simulink model "RuleBasedAlgo_sfunc_model"  (R2018b)
settings: Solver=ode2  StartTime=0.0  StopTime=inf  FixedStep=t_step  RelTol=1e-3
undefined symbols (not defined in the file or in its folder): A123_ESS, cs_ll, cs_ul
libraries: simulink x1
settings Model: Creator=Aman-Home  LastModifiedBy=Aman-Home

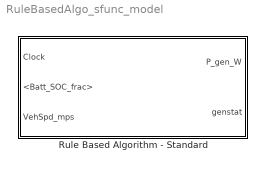
== system RuleBasedAlgo_sfunc_model ==
  Rule Based Algorithm - Standard : Subsystem

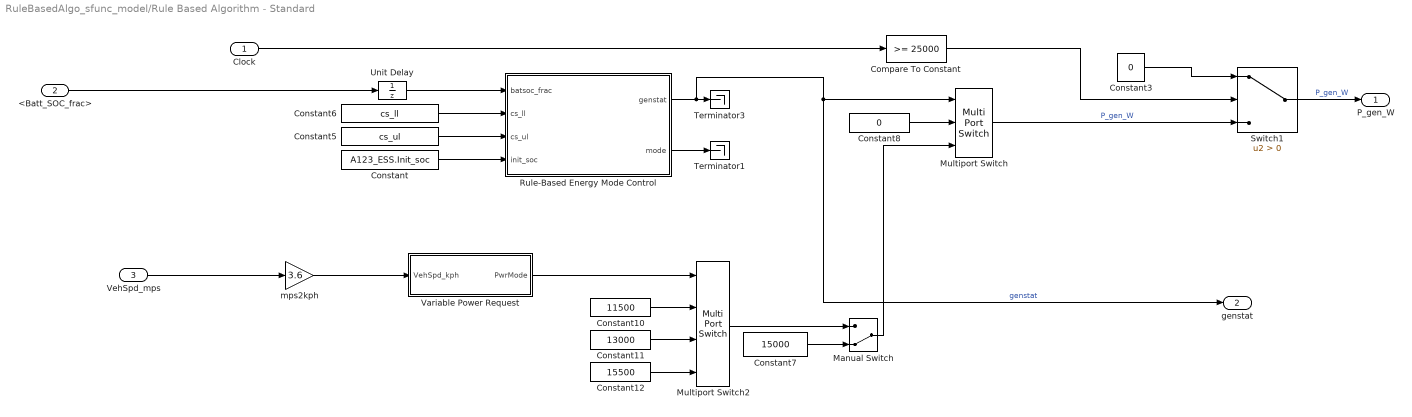
== system RuleBasedAlgo_sfunc_model/Rule Based Algorithm - Standard ==
  Clock : Inport
  <Batt_SOC_frac> : Inport  Port=2
  VehSpd_mps : Inport  Port=3
  Compare To Constant : simulink/Logic and Bit Operations/Compare To Constant  relop=>=  const=25000  OutDataTypeStr=boolean
  Constant : Constant  Value=A123_ESS.Init_soc
  Constant10 : Constant  Value=11500
  Constant11 : Constant  Value=13000
  Constant12 : Constant  Value=15500
  Constant3 : Constant  Value=0
  Constant5 : Constant  Value=cs_ul
  Constant6 : Constant  Value=cs_ll
  Constant7 : Constant  Value=15000
  Constant8 : Constant  Value=0
  Manual Switch : ManualSwitch  CurrentSetting=0
  Multiport Switch : MultiPortSwitch  DataPortOrder=Zero-based contiguous  Inputs=2  zeroidx=on
  Multiport Switch2 : MultiPortSwitch  DataPortOrder=Zero-based contiguous  zeroidx=on
  Rule-Based Energy Mode Control : Stateflow chart  TreatAsAtomicUnit=on
  Switch1 : Switch  Criteria=u2 > Threshold
  Terminator1 : Terminator
  Terminator3 : Terminator
  Unit Delay : UnitDelay  SampleTime=-1
  Variable Power Request : MATLAB Function  TreatAsAtomicUnit=on
  mps2kph : Gain  Gain=3.6
  P_gen_W : Outport
  genstat : Outport  Port=2
  wires:
  Multiport Switch2/1 -> Manual Switch/1
  Constant12/1 -> Multiport Switch2/4
  Constant11/1 -> Multiport Switch2/3
  Variable Power Request/1(PwrMode) -> Multiport Switch2/1
  Constant3/1 -> Switch1/1
  <Batt_SOC_frac>/1 -> Unit Delay/1
  Constant/1 -> Rule-Based Energy Mode Control/4(init_soc)
  Constant10/1 -> Multiport Switch2/2
  Constant8/1 -> Multiport Switch/2
  Clock/1 -> Compare To Constant/1
  Rule-Based Energy Mode Control/2(mode) -> Terminator1/1
  Constant7/1 -> Manual Switch/2
  Rule-Based Energy Mode Control/1(genstat) -> genstat/1, Multiport Switch/1, Terminator3/1  "genstat"
  VehSpd_mps/1 -> mps2kph/1
  Unit Delay/1 -> Rule-Based Energy Mode Control/1(batsoc_frac)
  mps2kph/1 -> Variable Power Request/1(VehSpd_kph)
  Constant5/1 -> Rule-Based Energy Mode Control/3(cs_ul)
  Compare To Constant/1 -> Switch1/2
  Multiport Switch/1 -> Switch1/3  "P_gen_W"
  Constant6/1 -> Rule-Based Energy Mode Control/2(cs_ll)
  Manual Switch/1 -> Multiport Switch/3
  Switch1/1 -> P_gen_W/1  "P_gen_W"

== stateflow chart RuleBasedAlgo_sfunc_model/Rule Based Algorithm - Standard/Rule-Based Energy Mode Control ==
  state Initialization
  state CDMode
    du:
    mode = 0;
    genstat = 0;
  state CSModeGen
    du:
    mode = 1;
    genstat = 1;
  state CSModeNoGen
    du:
    mode = 1;
    genstat = 0;
  (default) -> Initialization
  Initialization -> (junction 7) [order 1] : [batsoc_frac <= init_soc && ...
      | batsoc_frac >= cs_ll]
  Initialization -> (junction 10) [order 2] : [batsoc_frac < cs_ll]
  (junction 7) -> CDMode
  (junction 10) -> CSModeGen
  CDMode -> CSModeGen : [batsoc_frac < cs_ll]
  CSModeGen -> CSModeNoGen : [batsoc_frac >= cs_ul]
  CSModeNoGen -> CSModeGen : [batsoc_frac < cs_ll]
  data: batsoc_frac input; cs_ll input; cs_ul input; init_soc input; genstat output double; mode output double

== matlab function RuleBasedAlgo_sfunc_model/Rule Based Algorithm - Standard/Variable Power Request ==
  data: VehSpd_kph input; PwrMode output
function PwrMode = VarPwrReq(VehSpd_kph)
    if VehSpd_kph >= 0 && VehSpd_kph < 48
        PwrMode = 0;
    elseif VehSpd_kph >= 48 && VehSpd_kph < 97
        PwrMode = 1;
    else
        PwrMode = 2;
    end
end
